simulink model "steering"  (R2013b)
settings: Solver=ode45  StartTime=0.0  StopTime=10.0  RelTol=1e-3
values from neighbouring files (symbols this model uses):
  w_w = 250    [bla.m]
  w_z = 1.5    [bla.m]
settings Model: Creator=daniel  LastModifiedBy=daniel

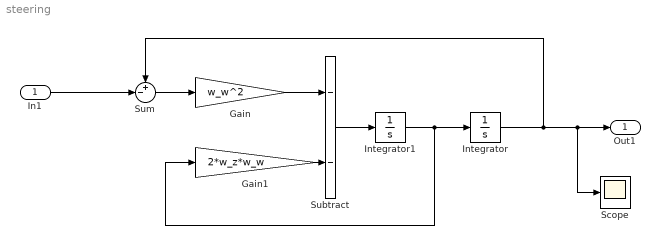
== system steering ==
  In1 : Inport
  Gain : Gain  Gain=w_w^2
  Gain1 : Gain  Gain=2*w_z*w_w
  Integrator : Integrator
  Integrator1 : Integrator
  Scope : Scope
  Subtract : Sum  Inputs=--
  Sum : Sum  Inputs=+-|
  Out1 : Outport
  wires:
  Integrator/1 -> Out1/1, Scope/1, Sum/1
  Subtract/1 -> Integrator1/1
  Sum/1 -> Gain/1
  Integrator1/1 -> Gain1/1, Integrator/1
  Gain/1 -> Subtract/1
  Gain1/1 -> Subtract/2
  In1/1 -> Sum/2
